simulink model "IC1"  (R2017b)
settings: Solver=FixedStepAuto  StartTime=0.0  StopTime=10.0  FixedStep=0.1  RelTol=1e-3
settings Model: Creator=hbourbou  LastModifiedBy=hbourbou

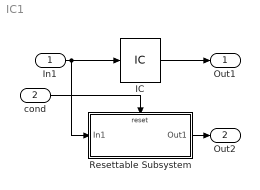
== system IC1 ==
  In1 : Inport
  cond : Inport  Port=2  OutDataTypeStr=boolean
  IC : InitialCondition  Value=1.2
  Resettable Subsystem : Subsystem  TreatAsAtomicUnit=on
  Out1 : Outport
  Out2 : Outport  Port=2
  wires:
  In1/1 -> Resettable Subsystem/1(In1), IC/1
  IC/1 -> Out1/1
  cond/1 -> Resettable Subsystem/Reset
  Resettable Subsystem/1(Out1) -> Out2/1

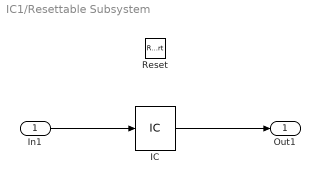
== system IC1/Resettable Subsystem ==
  In1 : Inport
  Reset : ResetPort  DisableCoverage=on  ResetTriggerType=either
  IC : InitialCondition  Value=1.2
  Out1 : Outport
  wires:
  In1/1 -> IC/1
  IC/1 -> Out1/1
